simulink model "main"  (R2022a)
settings: Solver=FixedStepAuto  StartTime=0.0  StopTime=10.0  FixedStep=0.01  RelTol=1e-3
undefined symbols (not defined in the file): CM, CT, d, sqrt22
libraries: simulink x2, shared6dof x1, vrlib x1
settings Model: Creator=Lenovo  LastModifiedBy=Lenovo
settings SolverCC: ZeroCrossControl=EnableAll
settings OptimizationCC: DefaultParameterBehavior=Inlined  EnhancedBackFolding=on  PassReuseOutputArgsAs=Individual arguments  ZeroExternalMemoryAtStartup=off  ZeroInternalMemoryAtStartup=off  OptimizeBlockOrder=speed  DifferentSizesBufferReuse=on  OptimizationCustomize=off  EfficientTunableParamExpr=on
settings DebuggingCC: ParameterTunabilityLossMsg=error
settings SFSimCC: MATLABDynamicMemAlloc=off
settings RTWCC: SystemTargetFile=ert.tlc  TemplateMakefile=ert_default_tmf
settings CodeAppCC: ForceParamTrailComments=on  IgnoreCustomStorageClasses=off  OperatorAnnotations=on  SimulinkDataObjDesc=on  SFDataObjDesc=on  InsertBlockDesc=on
settings ERTTargetCC: TargetLangStandard=C99 (ISO)  GenerateSampleERTMain=on  InlinedParameterPlacement=NonHierarchical  ERTCustomFileTemplate=example_file_process.tlc

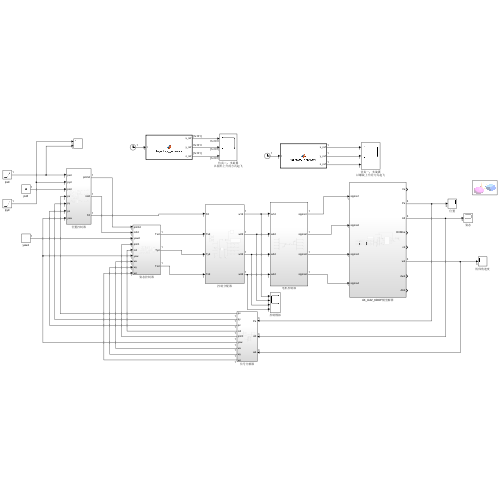
[thumbnail: Simulink's stored preview of the top-level diagram]
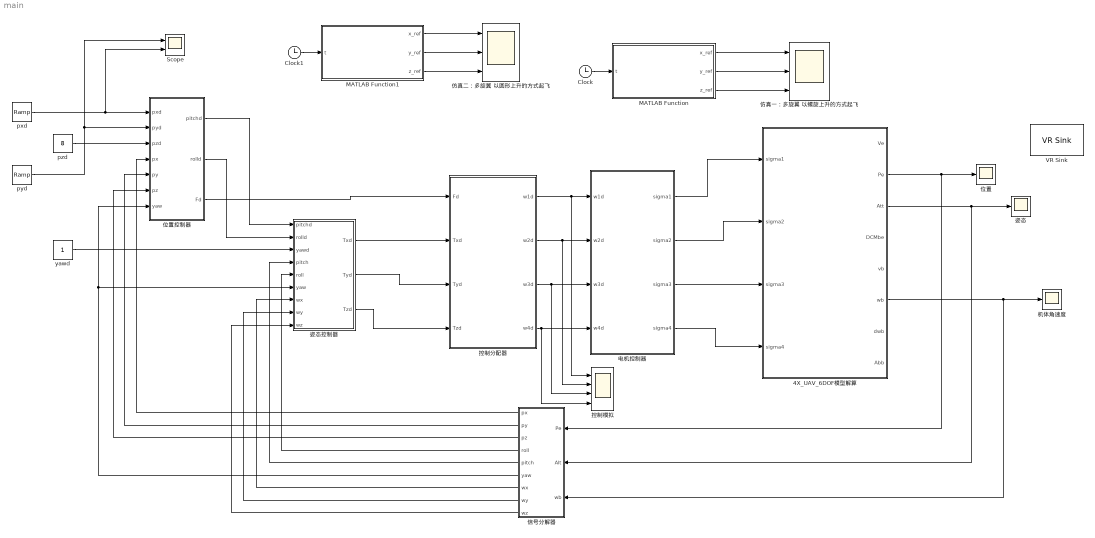
== system main ==
  4X_UAV_6DOF模型解算 : Subsystem
  Clock : Clock
  Clock1 : Clock
  MATLAB Function : MATLAB Function  TreatAsAtomicUnit=on
  MATLAB Function1 : MATLAB Function  TreatAsAtomicUnit=on
  Scope : Scope  NumInputPorts=2
  VR Sink : vrlib/VR Sink  InstantiateOnLoad=on  SampleTime=0.1  ViewEnable=on  RemoteChange=off  RemoteView=on  AutoView=off  VideoDimensions=[]  AllowVariableSize=off
  pxd : simulink/Sources/Ramp  slope=2  start=0  InitialOutput=0
  pyd : simulink/Sources/Ramp  slope=4  start=0  InitialOutput=0
  pzd : Constant  Value=8
  yawd : Constant
  仿真一：多旋翼 以螺旋上升的方式起飞 : Scope  NumInputPorts=3
  仿真二：多旋翼 以圆形上升的方式起飞 : Scope  NumInputPorts=3
  位置 : Scope
  位置控制器 : Subsystem
  信号分解器 : Subsystem
  姿态 : Scope
  姿态控制器 : Subsystem
  控制分配器 : Subsystem
  控制模拟 : Scope  NumInputPorts=4
  机体角速度 : Scope
  电机控制器 : Subsystem
  wires:
  pxd/1 -> Scope/2, 位置控制器/1(pxd)
  pyd/1 -> Scope/1, 位置控制器/2(pyd)
  pzd/1 -> 位置控制器/3(pzd)
  MATLAB Function/2(y_ref) -> 仿真一：多旋翼 以螺旋上升的方式起飞/2
  MATLAB Function/3(z_ref) -> 仿真一：多旋翼 以螺旋上升的方式起飞/3
  MATLAB Function/1(x_ref) -> 仿真一：多旋翼 以螺旋上升的方式起飞/1
  Clock/1 -> MATLAB Function/1(t)
  Clock1/1 -> MATLAB Function1/1(t)
  MATLAB Function1/1(x_ref) -> 仿真二：多旋翼 以圆形上升的方式起飞/1
  MATLAB Function1/3(z_ref) -> 仿真二：多旋翼 以圆形上升的方式起飞/3
  MATLAB Function1/2(y_ref) -> 仿真二：多旋翼 以圆形上升的方式起飞/2
  信号分解器/1(px) -> 位置控制器/4(px)
  信号分解器/2(py) -> 位置控制器/5(py)
  信号分解器/3(pz) -> 位置控制器/6(pz)
  信号分解器/6(yaw) -> 位置控制器/7(yaw), 姿态控制器/6(yaw)
  位置控制器/1(pitchd) -> 姿态控制器/1(pitchd)
  位置控制器/2(rolld) -> 姿态控制器/2(rolld)
  信号分解器/7(wx) -> 姿态控制器/7(wx)
  信号分解器/8(wy) -> 姿态控制器/8(wy)
  信号分解器/9(wz) -> 姿态控制器/9(wz)
  信号分解器/4(roll) -> 姿态控制器/5(roll)
  信号分解器/5(pitch) -> 姿态控制器/4(pitch)
  yawd/1 -> 姿态控制器/3(yawd)
  位置控制器/3(Fd) -> 控制分配器/1(Fd)
  姿态控制器/1(Txd) -> 控制分配器/2(Txd)
  姿态控制器/2(Tyd) -> 控制分配器/3(Tyd)
  姿态控制器/3(Tzd) -> 控制分配器/4(Tzd)
  控制分配器/1(w1d) -> 控制模拟/1, 电机控制器/1(w1d)
  控制分配器/2(w2d) -> 控制模拟/2, 电机控制器/2(w2d)
  控制分配器/3(w3d) -> 控制模拟/3, 电机控制器/3(w3d)
  控制分配器/4(w4d) -> 电机控制器/4(w4d), 控制模拟/4
  电机控制器/1(sigma1) -> 4X_UAV_6DOF模型解算/1(sigma1)
  电机控制器/2(sigma2) -> 4X_UAV_6DOF模型解算/2(sigma2)
  电机控制器/3(sigma3) -> 4X_UAV_6DOF模型解算/3(sigma3)
  电机控制器/4(sigma4) -> 4X_UAV_6DOF模型解算/4(sigma4)
  4X_UAV_6DOF模型解算/2(Pe) -> 信号分解器/1(Pe), 位置/1
  4X_UAV_6DOF模型解算/3(Att) -> 信号分解器/2(Alt), 姿态/1
  4X_UAV_6DOF模型解算/6(wb) -> 信号分解器/3(wb), 机体角速度/1

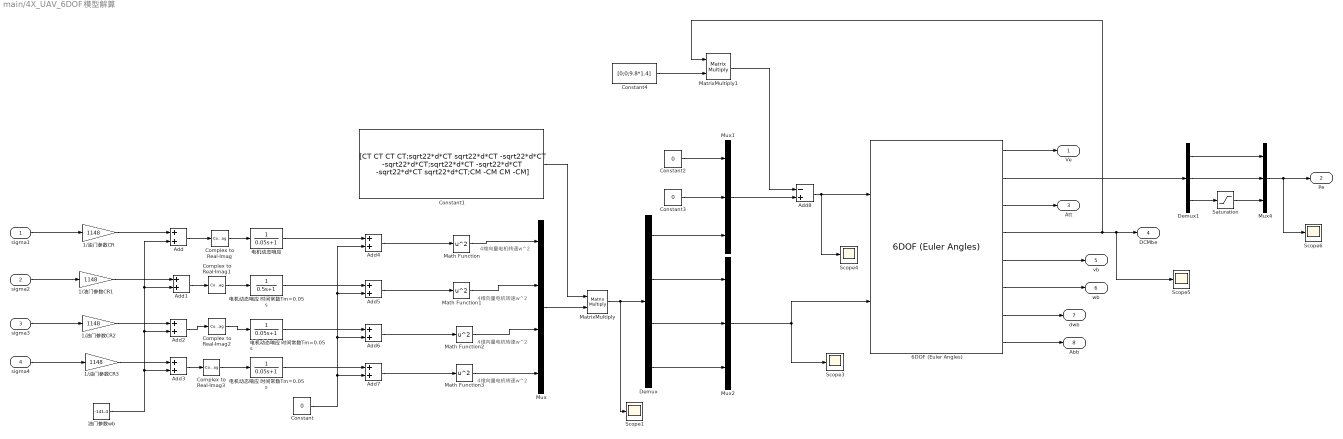
== system main/4X_UAV_6DOF模型解算 ==
  note: 4维向量电机转速w^2
  note: 4维向量电机转速w^2
  note: 4维向量电机转速w^2
  note: 4维向量电机转速w^2
  sigma1 : Inport
      settings: SignalType=complex
  sigma2 : Inport  Port=2
      settings: SignalType=complex
  sigma3 : Inport  Port=3
      settings: SignalType=complex
  sigma4 : Inport  Port=4
      settings: SignalType=complex
  1/油门参数CR{,1..3} (4 alike) : Gain  Gain=1148
  6DOF (Euler Angles) : shared6dof/6DOF (Euler Angles)  units=Metric (MKS)  mtype=Fixed  rep=Euler Angles  xme_0=[0 0 0]  Vm_0=[0 0 0]  eul_0=[0 0 0]  pm_0=[0 0 0]  mass_0=1.4  mass_e=0.5  mass_f=2.0  inertia=[0.0211,0,0;0,0.0219,0;0,0,0.0366]  inertia_e=eye(3)  inertia_f=2*eye(3)  k_quat=1.0  vre_flag=on  abi_flag=off  aMode=0  xme_statename=''  Vm_statename=''  eul_statename=''  quat_statename=''  pm_statename=''  mass_statename=''
      settings: SourceProductBaseCode=AE,PW,DR,MT,VE
  Add{,1..3} (4 alike) : Sum  AccumDataTypeStr=double  OutDataTypeStr=double
  Add{4..7} (4 alike) : Sum
  Add8 : Sum  Inputs=-+
  Complex to Real-Imag{,1..3} (4 alike) : ComplexToRealImag  Output=Real
  Constant : Constant  Value=0
  Constant1 : Constant  Value=[CT CT CT CT;sqrt22*d*CT sqrt22*d*CT -sqrt22*d*CT -sqrt22*d*CT;sqrt22*d*CT -sqrt22*d*CT -sqrt22*d*CT sqrt22*d*CT;CM -CM CM -CM]
  Constant2 : Constant  Value=0
  Constant3 : Constant  Value=0
  Constant4 : Constant  Value=[0;0;9.8*1.4]
  Demux : Demux
  Demux1 : Demux  Outputs=3
  Math Function{,1..3} (4 alike) : Math  Operator=square
  MatrixMultiply : Product  Multiplication=Matrix(*)
  MatrixMultiply1 : Product  Multiplication=Matrix(*)
  Mux : Mux
  Mux1 : Mux  Inputs=3
  Mux2 : Mux  Inputs=3
  Mux4 : Mux  Inputs=3
  Saturation : Saturate
  Scope{1,3..6} (5 alike) : Scope
  油门参数wb : Constant  Value=-141.4
  电机动态响应 : TransferFcn  Denominator=[0.05 1]
  电机动态响应 时间常数Tm=0.05s : TransferFcn  Denominator=[0.5 1]
  "电机动态响应 时间常数Tm=0.05s " : TransferFcn  Denominator=[0.05 1]
  电机动态响应 时间常数Tm=0.05s : TransferFcn  Denominator=[0.05 1]
  Ve : Outport
  Pe : Outport  Port=2
  Att : Outport  Port=3
  DCMbe : Outport  Port=4
  vb : Outport  Port=5
  wb : Outport  Port=6
  dwb : Outport  Port=7
  Abb : Outport  Port=8
  wires:
  6DOF (Euler Angles)/2 -> Demux1/1
  1/油门参数CR3/1 -> Add3/1
  Mux4/1 -> Pe/1, Scope6/1
  Add4/1 -> Math Function/1
  6DOF (Euler Angles)/4 -> DCMbe/1, Scope5/1, MatrixMultiply1/1
  油门参数wb/1 -> Add/2, Add1/2, Add2/2, Add3/2
  Add/1 -> Complex to Real-Imag/1
  1/油门参数CR/1 -> Add/1
  6DOF (Euler Angles)/5 -> vb/1
  Demux/3 -> Mux2/2
  6DOF (Euler Angles)/7 -> dwb/1
  6DOF (Euler Angles)/3 -> Att/1
  Demux1/3 -> Saturation/1
  sigma4/1 -> 1/油门参数CR3/1
  Demux1/1 -> Mux4/1
  Add8/1 -> 6DOF (Euler Angles)/1, Scope4/1
  Demux/1 -> Mux1/3
  6DOF (Euler Angles)/8 -> Abb/1
  Demux/4 -> Mux2/3
  电机动态响应 时间常数Tm=0.05s/1 -> Add7/1
  Mux/1 -> MatrixMultiply/2
  sigma3/1 -> 1/油门参数CR2/1
  Add5/1 -> Math Function1/1
  Add1/1 -> Complex to Real-Imag1/1
  6DOF (Euler Angles)/6 -> wb/1
  1/油门参数CR2/1 -> Add2/1
  1/油门参数CR1/1 -> Add1/1
  Saturation/1 -> Mux4/3
  Demux1/2 -> Mux4/2
  sigma2/1 -> 1/油门参数CR1/1
  Demux/2 -> Mux2/1
  电机动态响应 时间常数Tm=0.05s/1 -> Add5/1
  sigma1/1 -> 1/油门参数CR/1
  Math Function/1 -> Mux/1
  Mux2/1 -> Scope3/1, 6DOF (Euler Angles)/2
  Constant3/1 -> Mux1/2
  Constant2/1 -> Mux1/1
  6DOF (Euler Angles)/1 -> Ve/1
  MatrixMultiply1/1 -> Add8/1
  Constant4/1 -> MatrixMultiply1/2
  Constant/1 -> Add4/2, Add5/2, Add6/2, Add7/2
  "电机动态响应 时间常数Tm=0.05s "/1 -> Add6/1
  电机动态响应/1 -> Add4/1
  Add6/1 -> Math Function2/1
  Add2/1 -> Complex to Real-Imag2/1
  Add3/1 -> Complex to Real-Imag3/1
  Mux1/1 -> Add8/2
  MatrixMultiply/1 -> Demux/1, Scope1/1
  Math Function1/1 -> Mux/2
  Constant1/1 -> MatrixMultiply/1
  Math Function2/1 -> Mux/3
  Add7/1 -> Math Function3/1
  Math Function3/1 -> Mux/4
  Complex to Real-Imag/1 -> 电机动态响应/1
  Complex to Real-Imag1/1 -> 电机动态响应 时间常数Tm=0.05s/1
  Complex to Real-Imag2/1 -> "电机动态响应 时间常数Tm=0.05s "/1
  Complex to Real-Imag3/1 -> 电机动态响应 时间常数Tm=0.05s/1

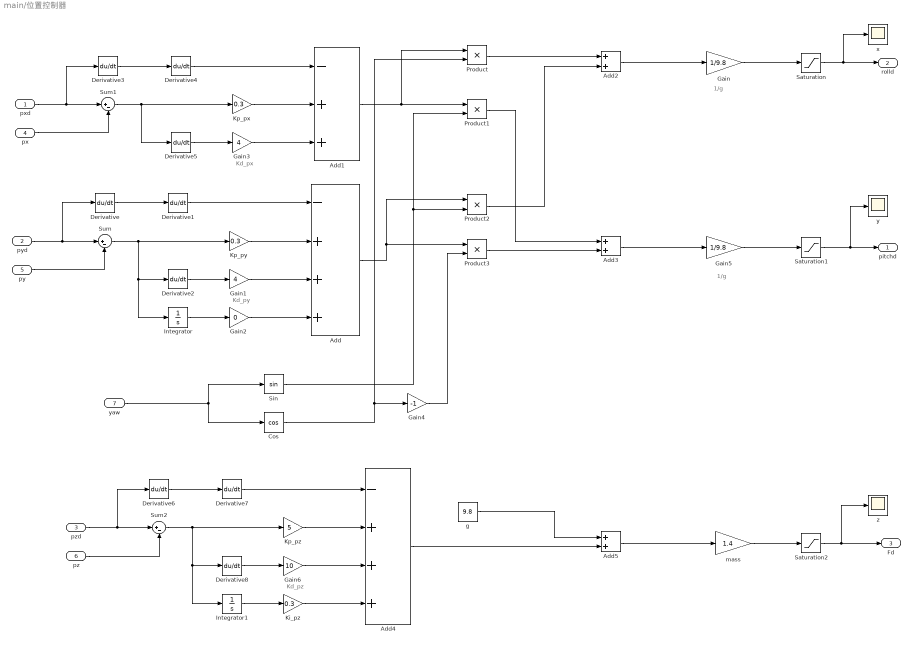
== system main/位置控制器 ==
  note: 1/g
  note: Kd_py
  note: Kd_px
  note: 1/g
  note: Kd_pz
  pxd : Inport
  pyd : Inport  Port=2
  pzd : Inport  Port=3
  px : Inport  Port=4
  py : Inport  Port=5
  pz : Inport  Port=6
  yaw : Inport  Port=7
  Add : Sum  Inputs=-+++
  Add1 : Sum  Inputs=-++
  Add2 : Sum
  Add3 : Sum
  Add4 : Sum  Inputs=-+++
  Add5 : Sum
  Cos : Trigonometry  Operator=cos
  Derivative{,1..8} (9 alike) : Derivative
  Gain : Gain  Gain=1/9.8
  Gain1 : Gain  Gain=4
  Gain2 : Gain  Gain=0
  Gain3 : Gain  Gain=4
  Gain4 : Gain  Gain=-1
  Gain5 : Gain  Gain=1/9.8
  Gain6 : Gain  Gain=10
  Integrator : Integrator
  Integrator1 : Integrator
  Ki_pz : Gain  Gain=0.3
  Kp_px : Gain  Gain=0.3
  Kp_py : Gain  Gain=0.3
  Kp_pz : Gain  Gain=5
  Product{,1..3} (4 alike) : Product
  Saturation : Saturate
  Saturation1 : Saturate
  Saturation2 : Saturate
  Sin : Trigonometry
  Sum : Sum  Inputs=|+-
  Sum1 : Sum  Inputs=|+-
  Sum2 : Sum  Inputs=|+-
  g : Constant  Value=9.8
  mass : Gain  Gain=1.4
  x : Scope
  y : Scope
  z : Scope
  pitchd : Outport
  rolld : Outport  Port=2
  Fd : Outport  Port=3
  wires:
  Sum/1 -> Derivative2/1, Integrator/1, Kp_py/1
  Cos/1 -> Gain4/1, Product/2
  Derivative2/1 -> Gain1/1
  Gain6/1 -> Add4/3
  px/1 -> Sum1/2
  pyd/1 -> Derivative/1, Sum/1
  Saturation/1 -> rolld/1, x/1
  Add1/1 -> Product/1, Product1/1
  Derivative6/1 -> Derivative7/1
  Derivative/1 -> Derivative1/1
  Add/1 -> Product2/1, Product3/1
  Saturation1/1 -> pitchd/1, y/1
  pz/1 -> Sum2/2
  g/1 -> Add5/1
  Add2/1 -> Gain/1
  Kp_px/1 -> Add1/2
  Add3/1 -> Gain5/1
  Gain5/1 -> Saturation1/1
  Derivative3/1 -> Derivative4/1
  Product2/1 -> Add2/2
  Integrator/1 -> Gain2/1
  Derivative5/1 -> Gain3/1
  Gain/1 -> Saturation/1
  Integrator1/1 -> Ki_pz/1
  Gain1/1 -> Add/3
  Kp_py/1 -> Add/2
  Derivative4/1 -> Add1/1
  Ki_pz/1 -> Add4/4
  Kp_pz/1 -> Add4/2
  Derivative1/1 -> Add/1
  Product3/1 -> Add3/2
  Product1/1 -> Add3/1
  Sum1/1 -> Kp_px/1, Derivative5/1
  pzd/1 -> Derivative6/1, Sum2/1
  Sin/1 -> Product2/2, Product1/2
  Gain4/1 -> Product3/2
  Sum2/1 -> Integrator1/1, Derivative8/1, Kp_pz/1
  Product/1 -> Add2/1
  yaw/1 -> Cos/1, Sin/1
  Add4/1 -> Add5/2
  py/1 -> Sum/2
  Gain2/1 -> Add/4
  mass/1 -> Saturation2/1
  Derivative7/1 -> Add4/1
  Gain3/1 -> Add1/3
  Add5/1 -> mass/1
  Saturation2/1 -> Fd/1, z/1
  pxd/1 -> Sum1/1, Derivative3/1
  Derivative8/1 -> Gain6/1

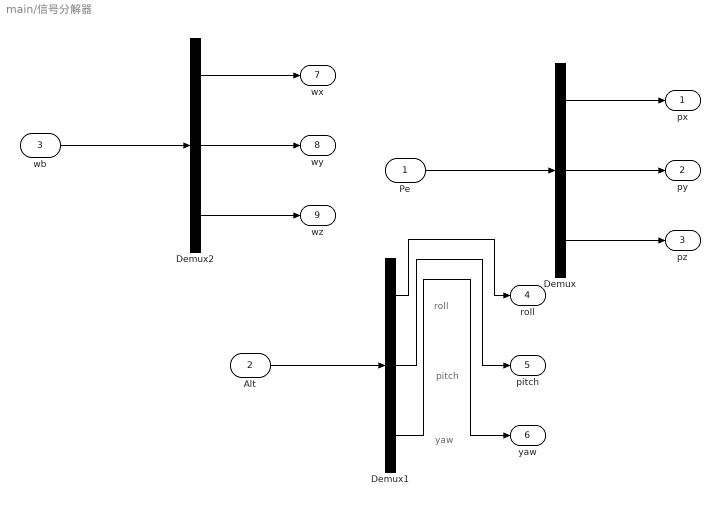
== system main/信号分解器 ==
  note: yaw
  note: pitch
  note: roll
  Pe : Inport
  Alt : Inport  Port=2
  wb : Inport  Port=3
  Demux : Demux  Outputs=3
  Demux1 : Demux  Outputs=3
  Demux2 : Demux  Outputs=3
  px : Outport
  py : Outport  Port=2
  pz : Outport  Port=3
  roll : Outport  Port=4
  pitch : Outport  Port=5
  yaw : Outport  Port=6
  wx : Outport  Port=7
  wy : Outport  Port=8
  wz : Outport  Port=9
  wires:
  Demux1/2 -> pitch/1
  Demux/3 -> pz/1
  Demux2/1 -> wx/1
  Demux/2 -> py/1
  Demux1/1 -> roll/1
  Pe/1 -> Demux/1
  Demux1/3 -> yaw/1
  Demux2/3 -> wz/1
  Demux2/2 -> wy/1
  Alt/1 -> Demux1/1
  wb/1 -> Demux2/1
  Demux/1 -> px/1

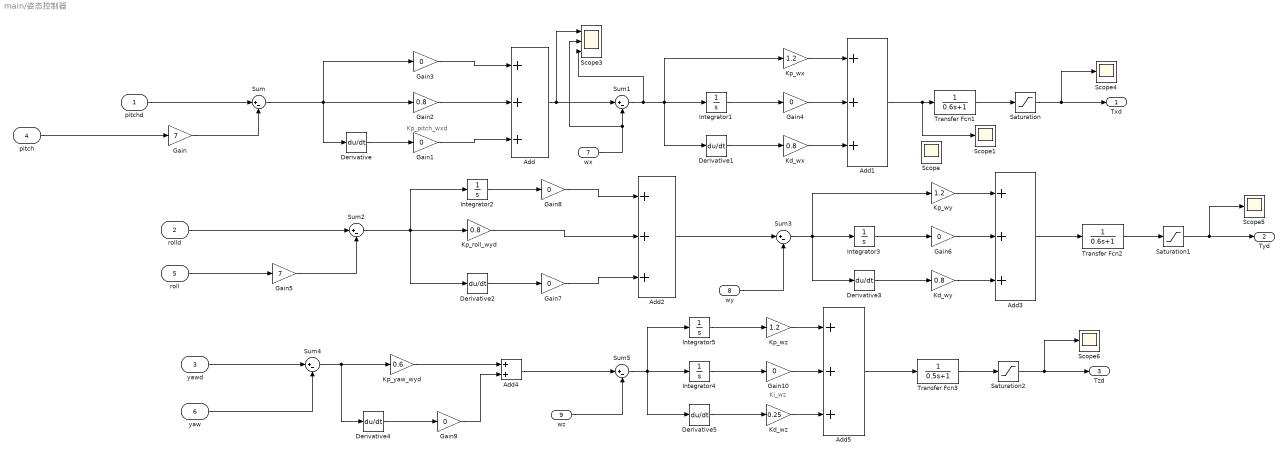
== system main/姿态控制器 ==
  note: Ki_wz
  note: Kp_pitch_wxd
  pitchd : Inport
  rolld : Inport  Port=2
  yawd : Inport  Port=3
  pitch : Inport  Port=4
  roll : Inport  Port=5
  yaw : Inport  Port=6
  wx : Inport  Port=7
  wy : Inport  Port=8
  wz : Inport  Port=9
  Add{,1..3,5} (5 alike) : Sum  Inputs=+++
  Add4 : Sum
  Derivative{,1..5} (6 alike) : Derivative
  Gain : Gain  Gain=7
  Gain{1,3..4,6..10} (8 alike) : Gain  Gain=0
  Gain2 : Gain  Gain=0.8
  Gain5 : Gain  Gain=7
  Integrator{1..5} (5 alike) : Integrator
  Kd_wx : Gain  Gain=0.8
  Kd_wy : Gain  Gain=0.8
  Kd_wz : Gain  Gain=0.25
  Kp_roll_wyd : Gain  Gain=0.8
  Kp_wx : Gain  Gain=1.2
  Kp_wy : Gain  Gain=1.2
  Kp_wz : Gain  Gain=1.2
  Kp_yaw_wyd : Gain  Gain=0.6
  Saturation : Saturate
  Saturation1 : Saturate
  Saturation2 : Saturate
  Scope{,1,4..6} (5 alike) : Scope
  Scope3 : Scope  NumInputPorts=3
  Sum{,1..5} (6 alike) : Sum  Inputs=|+-
  Transfer Fcn1 : TransferFcn  Numerator=[1 ]  Denominator=[0.6 1]
  Transfer Fcn2 : TransferFcn  Denominator=[0.6 1]
  Transfer Fcn3 : TransferFcn  Denominator=[0.5 1]
  Txd : Outport
  Tyd : Outport  Port=2
  Tzd : Outport  Port=3
  wires:
  Derivative1/1 -> Kd_wx/1
  Gain/1 -> Sum/2
  Saturation2/1 -> Tzd/1, Scope6/1
  Kd_wx/1 -> Add1/3
  Kd_wz/1 -> Add5/3
  Kp_wx/1 -> Add1/1
  Derivative5/1 -> Kd_wz/1
  Sum1/1 -> Integrator1/1, Kp_wx/1, Derivative1/1, Scope3/3
  Sum/1 -> Gain3/1, Derivative/1, Gain2/1
  Kp_wz/1 -> Add5/1
  Integrator1/1 -> Gain4/1
  Gain4/1 -> Add1/2
  Gain9/1 -> Add4/2
  Sum5/1 -> Integrator4/1, Integrator5/1, Derivative5/1
  pitchd/1 -> Sum/1
  Derivative/1 -> Gain1/1
  Sum4/1 -> Kp_yaw_wyd/1, Derivative4/1
  Gain10/1 -> Add5/2
  Add/1 -> Sum1/1, Scope3/1
  Gain3/1 -> Add/1
  Integrator2/1 -> Gain8/1
  Saturation/1 -> Txd/1, Scope4/1
  Gain2/1 -> Add/2
  Add4/1 -> Sum5/1
  Gain1/1 -> Add/3
  Derivative3/1 -> Kd_wy/1
  wx/1 -> Sum1/2, Scope3/2
  Transfer Fcn3/1 -> Saturation2/1
  yawd/1 -> Sum4/1
  pitch/1 -> Gain/1
  Sum3/1 -> Derivative3/1, Kp_wy/1, Integrator3/1
  rolld/1 -> Sum2/1
  Kp_roll_wyd/1 -> Add2/2
  Gain5/1 -> Sum2/2
  wy/1 -> Sum3/2
  Integrator4/1 -> Gain10/1
  Transfer Fcn1/1 -> Saturation/1
  Add5/1 -> Transfer Fcn3/1
  wz/1 -> Sum5/2
  roll/1 -> Gain5/1
  Derivative4/1 -> Gain9/1
  Gain7/1 -> Add2/3
  Kp_yaw_wyd/1 -> Add4/1
  yaw/1 -> Sum4/2
  Add3/1 -> Transfer Fcn2/1
  Integrator3/1 -> Gain6/1
  Kp_wy/1 -> Add3/1
  Kd_wy/1 -> Add3/3
  Gain6/1 -> Add3/2
  Transfer Fcn2/1 -> Saturation1/1
  Gain8/1 -> Add2/1
  Saturation1/1 -> Tyd/1, Scope5/1
  Sum2/1 -> Kp_roll_wyd/1, Integrator2/1, Derivative2/1
  Derivative2/1 -> Gain7/1
  Add2/1 -> Sum3/1
  Integrator5/1 -> Kp_wz/1
  Add1/1 -> Scope1/1, Transfer Fcn1/1

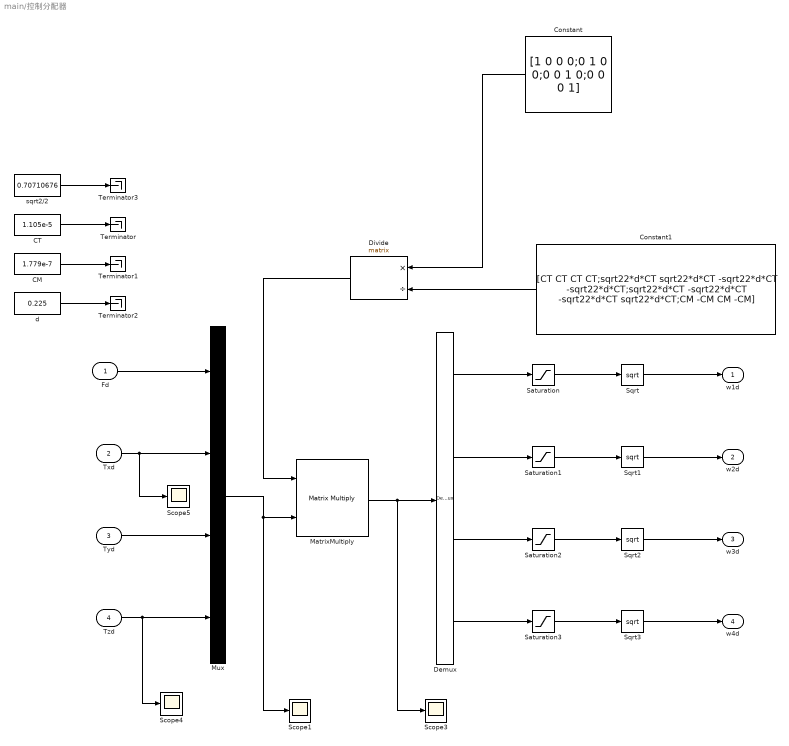
== system main/控制分配器 ==
  Fd : Inport
  Txd : Inport  Port=2
  Tyd : Inport  Port=3
  Tzd : Inport  Port=4
  CM : Constant  Value=1.779e-7
  CT : Constant  Value=1.105e-5
  Constant : Constant  Value=[1 0 0 0;0 1 0 0;0 0 1 0;0 0 0 1]
  Constant1 : Constant  Value=[CT CT CT CT;sqrt22*d*CT sqrt22*d*CT -sqrt22*d*CT -sqrt22*d*CT;sqrt22*d*CT -sqrt22*d*CT -sqrt22*d*CT sqrt22*d*CT;CM -CM CM -CM]
  Demux : Demux
  Divide : Product  Inputs=*/  Multiplication=Matrix(*)
  MatrixMultiply : Product  Multiplication=Matrix(*)  RndMeth=Nearest
  Mux : Mux
  Saturation{,1..3} (4 alike) : Saturate
  Scope{1,3..5} (4 alike) : Scope
  Sqrt{,1..3} (4 alike) : Sqrt  OutputSignalType=complex
  Terminator{,1..3} (4 alike) : Terminator
  d : Constant  Value=0.225
  sqrt2/2 : Constant  Value=0.70710676
  w1d : Outport
      settings: SignalType=complex
  w2d : Outport  Port=2
      settings: SignalType=complex
  w3d : Outport  Port=3
      settings: SignalType=complex
  w4d : Outport  Port=4
      settings: SignalType=complex
  wires:
  Sqrt1/1 -> w2d/1
  Constant/1 -> Divide/1
  MatrixMultiply/1 -> Demux/1, Scope3/1
  Sqrt/1 -> w1d/1
  Constant1/1 -> Divide/2
  Txd/1 -> Mux/2, Scope5/1
  Demux/3 -> Saturation2/1
  Saturation1/1 -> Sqrt1/1
  Divide/1 -> MatrixMultiply/1
  Sqrt3/1 -> w4d/1
  Demux/4 -> Saturation3/1
  Mux/1 -> MatrixMultiply/2, Scope1/1
  Demux/2 -> Saturation1/1
  CM/1 -> Terminator1/1
  Saturation/1 -> Sqrt/1
  Saturation3/1 -> Sqrt3/1
  Tyd/1 -> Mux/3
  Saturation2/1 -> Sqrt2/1
  Fd/1 -> Mux/1
  Sqrt2/1 -> w3d/1
  Demux/1 -> Saturation/1
  d/1 -> Terminator2/1
  sqrt2/2/1 -> Terminator3/1
  CT/1 -> Terminator/1
  Tzd/1 -> Mux/4, Scope4/1

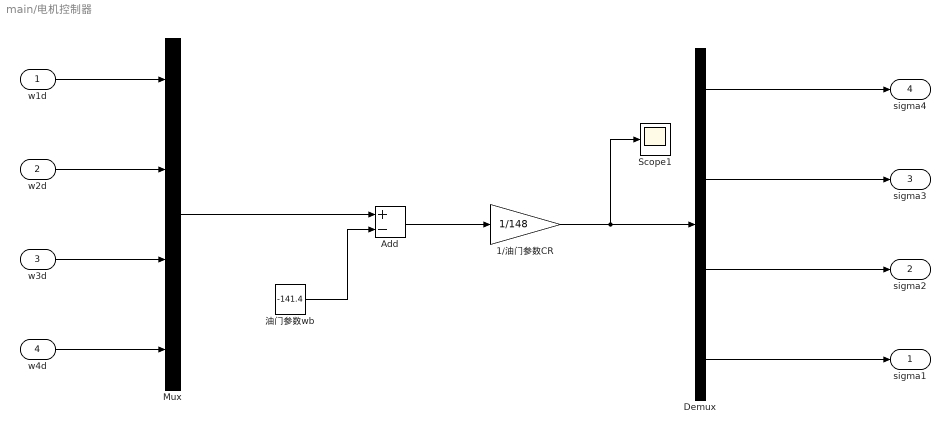
== system main/电机控制器 ==
  w1d : Inport
      settings: SignalType=complex
  w2d : Inport  Port=2
      settings: SignalType=complex
  w3d : Inport  Port=3
      settings: SignalType=complex
  w4d : Inport  Port=4
      settings: SignalType=complex
  1/油门参数CR : Gain  Gain=1/148
  Add : Sum  Inputs=+-
  Demux : Demux
  Mux : Mux
  Scope1 : Scope
  油门参数wb : Constant  Value=-141.4
  sigma1 : Outport
  sigma2 : Outport  Port=2
  sigma3 : Outport  Port=3
  sigma4 : Outport  Port=4
  wires:
  w1d/1 -> Mux/1
  Add/1 -> 1/油门参数CR/1
  Demux/3 -> sigma2/1
  1/油门参数CR/1 -> Demux/1, Scope1/1
  Demux/4 -> sigma1/1
  w3d/1 -> Mux/3
  Demux/1 -> sigma4/1
  Demux/2 -> sigma3/1
  w2d/1 -> Mux/2
  w4d/1 -> Mux/4
  油门参数wb/1 -> Add/2
  Mux/1 -> Add/1

== matlab function main/MATLAB Function ==
  data: t input; x_ref output; y_ref output; z_ref output
function [x_ref, y_ref, z_ref] = trajectory_generator(t)
    % 螺旋上升轨迹
    x_ref = 5 * cos(t);
    y_ref = 5 * sin(t);
    z_ref = 0.5 * t;
end

== matlab function main/MATLAB Function1 ==
  data: t input; x_ref output; y_ref output; z_ref output
function [x_ref, y_ref, z_ref] = trajectory_generator(t)
% 示例：生成圆形轨迹
t = 0:0.1:10;
x_ref = 5*cos(t);
y_ref = 5*sin(t);
z_ref = 2*t;
end
